simulink model "Simulink"  (R2020a)
settings: Solver=VariableStepAuto  StartTime=0.0  StopTime=600  RelTol=1e-3
settings Model: Creator=carlo  LastModifiedBy=carlo

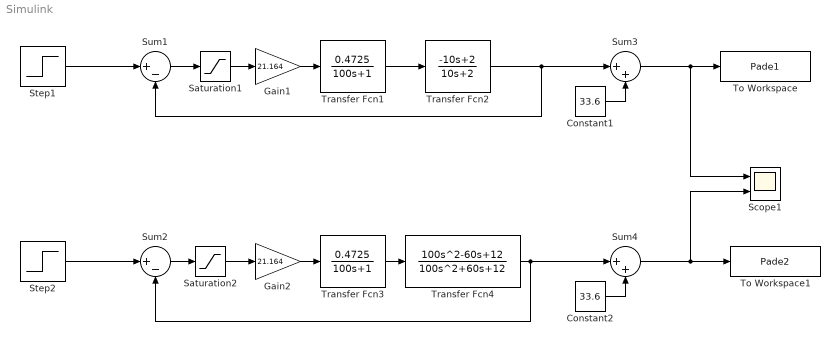
== system Simulink ==
  Constant1 : Constant  Value=33.6
  Constant2 : Constant  Value=33.6
  Gain1 : Gain  Gain=21.164
  Gain2 : Gain  Gain=21.164
  Saturation1 : Saturate  UpperLimit=24  LowerLimit=0
  Saturation2 : Saturate  UpperLimit=24  LowerLimit=0
  Scope1 : Scope  NumInputPorts=2
  Step1 : Step  After=11.4  SampleTime=0
  Step2 : Step  After=11.4  SampleTime=0
  Sum1 : Sum  Inputs=|+-
  Sum2 : Sum  Inputs=|+-
  Sum3 : Sum  Inputs=|++
  Sum4 : Sum  Inputs=|++
  To Workspace : ToWorkspace  VariableName=Pade1  SaveFormat=Timeseries  SampleTime=-1
  To Workspace1 : ToWorkspace  VariableName=Pade2  SaveFormat=Timeseries  SampleTime=-1
  Transfer Fcn1 : TransferFcn  Numerator=[0.4725]  Denominator=[100 1]
  Transfer Fcn2 : TransferFcn  Numerator=[-10 2]  Denominator=[10 2]
  Transfer Fcn3 : TransferFcn  Numerator=[0.4725]  Denominator=[100 1]
  Transfer Fcn4 : TransferFcn  Numerator=[100 -60 12]  Denominator=[100 60 12]
  wires:
  Constant1/1 -> Sum3/2
  Sum1/1 -> Saturation1/1
  Transfer Fcn1/1 -> Transfer Fcn2/1
  Gain1/1 -> Transfer Fcn1/1
  Transfer Fcn2/1 -> Sum1/2, Sum3/1
  Constant2/1 -> Sum4/2
  Sum2/1 -> Saturation2/1
  Transfer Fcn3/1 -> Transfer Fcn4/1
  Step2/1 -> Sum2/1
  Saturation2/1 -> Gain2/1
  Transfer Fcn4/1 -> Sum4/1, Sum2/2
  Gain2/1 -> Transfer Fcn3/1
  Step1/1 -> Sum1/1
  Sum3/1 -> To Workspace/1, Scope1/1
  Saturation1/1 -> Gain1/1
  Sum4/1 -> To Workspace1/1, Scope1/2
